simulink model "q3_a"  (R2016a)
settings: Solver=ode3  StartTime=0.0  StopTime=50  FixedStep=0.001  RelTol=1e-3
settings Model: Creator=Ahmet Asım  LastModifiedBy=Ahmet Asım

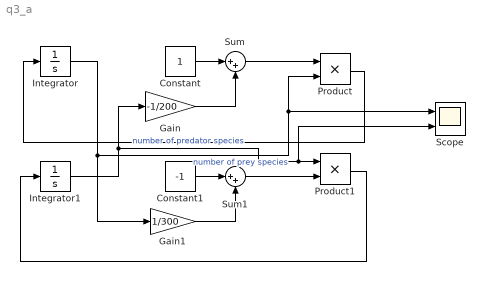
== system q3_a ==
  Constant : Constant
  Constant1 : Constant  Value=-1
  Gain : Gain  Gain=-1/200
  Gain1 : Gain  Gain=1/300
  Integrator : Integrator  InitialCondition=400
  Integrator1 : Integrator  InitialCondition=100
  Product : Product
  Product1 : Product
  Scope : Scope  NumInputPorts=2
  Sum : Sum  Inputs=|++
  Sum1 : Sum  Inputs=|++
  wires:
  Gain/1 -> Sum/2
  Constant/1 -> Sum/1
  Sum/1 -> Product/1
  Constant1/1 -> Sum1/1
  Gain1/1 -> Sum1/2
  Sum1/1 -> Product1/2
  Integrator1/1 -> Scope/2, Product1/1, Gain/1  "number of predator species"
  Integrator/1 -> Scope/1, Product/2, Gain1/1  "number of prey species"
  Product/1 -> Integrator/1
  Product1/1 -> Integrator1/1
